simulink model "monitoring_scheme"  (R2021b)
settings: Solver=VariableStepAuto  StartTime=0.0  StopTime=inf  RelTol=1e-3
libraries: instrumentseriallib x2
settings Model: Creator=popov  LastModifiedBy=popov

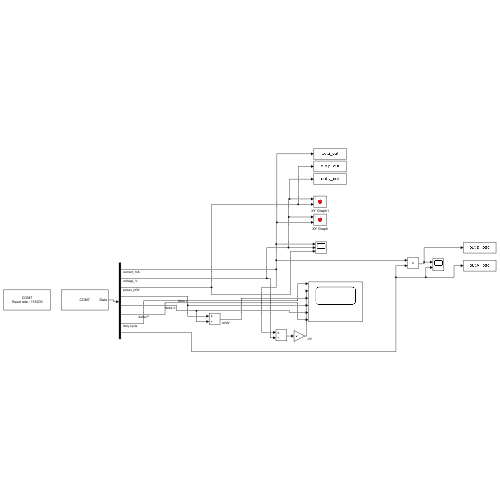
[thumbnail: Simulink's stored preview of the top-level diagram]
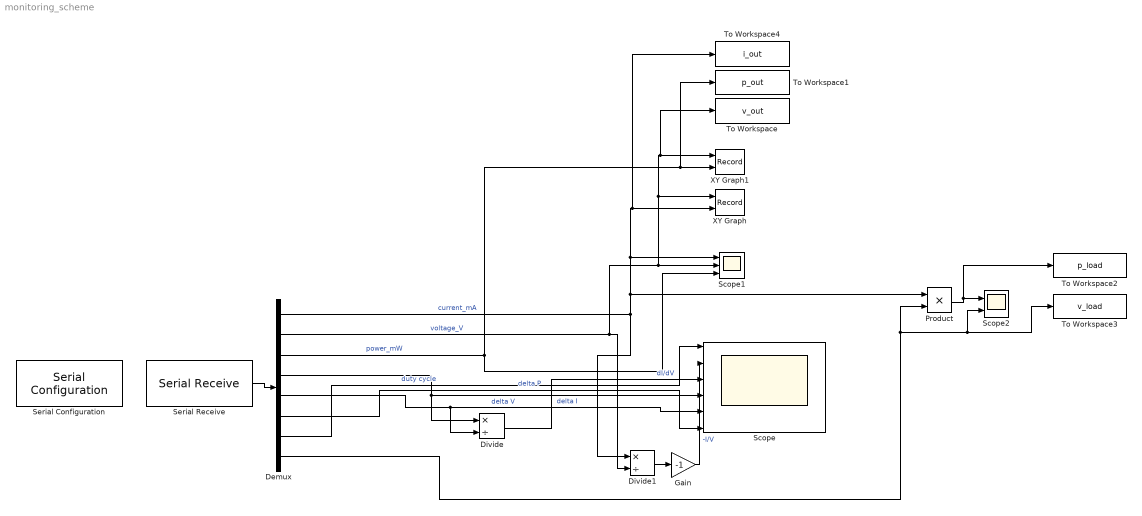
== system monitoring_scheme ==
  Demux : Demux  Outputs=8
  Divide : Product  Inputs=*/
  Divide1 : Product  Inputs=*/
  Gain : Gain  Gain=-1
  Product : Product
  Scope : Scope  NumInputPorts=6
  Scope1 : Scope  NumInputPorts=3
  Scope2 : Scope  NumInputPorts=2
  Serial Configuration : instrumentseriallib/Serial Configuration  Priority=-200000  Port=COM7  ComPort=COM7  BaudRate=115200  DataBits=8  Parity=none  StopBits=1  ByteOrder=little-endian  FlowControl=none  Timeout=10  SimulateUsing=Interpreted execution  BlockInModel=on
  Serial Receive : instrumentseriallib/Serial Receive  Priority=1  Port=COM7  ComPort=COM7  DataType=single  SaveDataType=uint8  ToggleHeader=on  Header=['N' 'N' 'N' 'N']  ToggleTerminator=on  Terminator=Custom terminator  CustomTerminator=['E' 'E' 'E' 'E']  ToggleDataSize=on  DataSize=[1 8]  EnableBlockingMode=on  ActionDataUnavailable=Output last received value  ActionWhenDataUnavailable=Output last received value  CustomValue=0  SampleTime=0.01  SimulateUsing=Interpreted execution  BlockInModel=on
  To Workspace : ToWorkspace  VariableName=v_out  SampleTime=-1
  To Workspace1 : ToWorkspace  VariableName=p_out  SampleTime=-1
  To Workspace2 : ToWorkspace  VariableName=p_load  SampleTime=-1
  To Workspace3 : ToWorkspace  VariableName=v_load  SaveFormat=Timeseries  SampleTime=-1
  To Workspace4 : ToWorkspace  VariableName=i_out  SampleTime=-1
  XY Graph : Record  FileSettingsInternal="{\"entries\":[{\"content\":{\"excelSettings\":{\"content\":{},\"type\":\"Streamout.ExcelSettings\"}},\"type\":\"Streamout.FileSettingStorage\",\"uuid\":\"80655a95-84e9-46a0-9290-fc7a58679d06\"}],\"packageUris\":[\"http://schema.mathworks.com/mf0/streamout_blocks/R2020a\"],\"version\":\"1.0\"}"  Layout=[1 1]  SignalsInternal="{\"entries\":[{\"content\":{\"signals\":[{\"content\":{\"blockPath\":[\"monitoring_scheme/XY Graph\"],\"channel\":[],\"dimensions\":[1,1],\"domain\":\"monitoring_scheme/XY Graph\",\"lineColor\":\"#a2142f\",\"plots\":[1],\"port\":1,\"sid\":[\"\"],\"signalID\":339801,\"signalName\":\"voltage_V\"},\"type\":\"RecordBlkView.Signal\",\"uuid\":\"68338ab6-0ca8-459b-94f8-0c80448d00af\"},{\"content\":{\"blockPath\":[\"monitoring_scheme/XY Graph\"],\"channel\":[],\"dimensions\":[1,1],\"domain\":\"monitoring_scheme/XY Graph\",\"lineColor\":\"#139fff\",\"plots\":[1],\"port\":2,\"sid\":[\"\"],\"signalID\":339805,\"signalName\":\"current_mA\"},\"type\":\"RecordBlkView.Signal\",\"uuid\":\"641f4f97-7725-40d3-b2a1-72f0798c3917\"}]},\"type\":\"RecordBlkView.InputSignals\",\"uuid\":\"c4b8f1f9-e6d4-410a-9d97-e36f87fb6d43\"}],\"packageUris\":[\"http://schema.mathworks.com/mf0/streamout_blocks/R2020a\"],\"version\":\"1.0\"}"  VisualizationBindings="{\"xyplotplugin\":{\"info\":[{\"series\":[{\"bindingParametersList\":[{\"parameter\":\"X-Axis\",\"signalID\":339801,\"signalName\":\"voltage_V\"},{\"parameter\":\"Y-Axis\",\"signalID\":339805,\"signalName\":\"current_mA\"}],\"seriesID\":60806}],\"subplotID\":1}]}}"  CompatibilityTag=XY
  XY Graph1 : Record  FileSettingsInternal="{\"entries\":[{\"content\":{\"excelSettings\":{\"content\":{},\"type\":\"Streamout.ExcelSettings\"}},\"type\":\"Streamout.FileSettingStorage\",\"uuid\":\"503910e1-a809-4fa5-aed5-c88c97986ab5\"}],\"packageUris\":[\"http://schema.mathworks.com/mf0/streamout_blocks/R2020a\"],\"version\":\"1.0\"}"  Layout=[1 1]  SignalsInternal="{\"entries\":[{\"content\":{\"signals\":[{\"content\":{\"blockPath\":[\"monitoring_scheme/XY Graph1\"],\"channel\":[],\"dimensions\":[1,1],\"domain\":\"monitoring_scheme/XY Graph1\",\"lineColor\":\"#a2142f\",\"plots\":[1],\"port\":1,\"sid\":[\"\"],\"signalID\":339809,\"signalName\":\"voltage_V\"},\"type\":\"RecordBlkView.Signal\",\"uuid\":\"bf2cd0b0-d0ea-463c-9563-3a25baf85463\"},{\"content\":{\"blockPath\":[\"monitoring_scheme/XY Graph1\"],\"channel\":[],\"dimensions\":[1,1],\"domain\":\"monitoring_scheme/XY Graph1\",\"lineColor\":\"#139fff\",\"plots\":[1],\"port\":2,\"sid\":[\"\"],\"signalID\":339813,\"signalName\":\"power_mW\"},\"type\":\"RecordBlkView.Signal\",\"uuid\":\"fa6cf987-0db4-4cf7-990e-fd8a35c9f405\"}]},\"type\":\"RecordBlkView.InputSignals\",\"uuid\":\"b5fc8b9f-e569-4f97-bbcd-77ad83b9a0a7\"}],\"packageUris\":[\"http://schema.mathworks.com/mf0/streamout_blocks/R2020a\"],\"version\":\"1.0\"}"  VisualizationBindings="{\"xyplotplugin\":{\"info\":[{\"series\":[{\"bindingParametersList\":[{\"parameter\":\"X-Axis\",\"signalID\":339809,\"signalName\":\"voltage_V\"},{\"parameter\":\"Y-Axis\",\"signalID\":339813,\"signalName\":\"power_mW\"}],\"seriesID\":44142}],\"subplotID\":1}]}}"  CompatibilityTag=XY
  wires:
  Serial Receive/1 -> Demux/1
  Demux/1 -> Product/1, To Workspace4/1, XY Graph/2, Scope1/1, Divide1/1  "current_mA"
  Demux/2 -> To Workspace/1, XY Graph1/1, XY Graph/1, Scope1/2, Divide1/2  "voltage_V"
  Demux/3 -> Scope1/3, To Workspace1/1, XY Graph1/2  "power_mW"
  Demux/4 -> Scope/4, Divide/1  "delta I"
  Demux/5 -> Scope/5, Divide/2  "delta V"
  Demux/6 -> Scope/6  "delta P"
  Divide1/1 -> Gain/1
  Divide/1 -> Scope/3  "dI/dV"
  Gain/1 -> Scope/2  "-I/V"
  Demux/7 -> Scope/1  "duty cycle"
  Demux/8 -> To Workspace3/1, Scope2/2, Product/2
  Product/1 -> To Workspace2/1, Scope2/1
